simulink model "task_1"  (R2024a)
settings: Solver=VariableStepAuto  StartTime=0.0  StopTime=10  RelTol=1e-3
undefined symbols (not defined in the file): a0, a1, a2, idy, iy, k0, k1
settings Model: Creator=kit  LastModifiedBy=kit

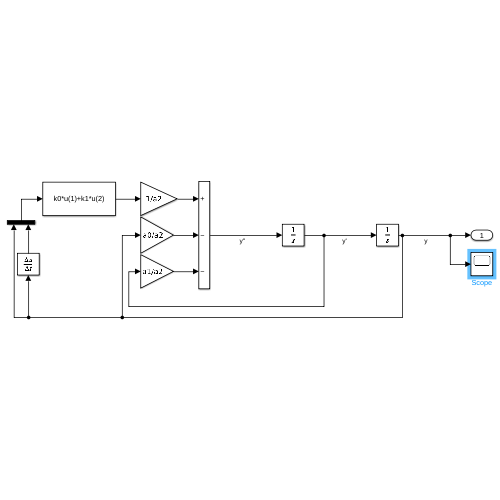
[thumbnail: Simulink's stored preview of the top-level diagram]
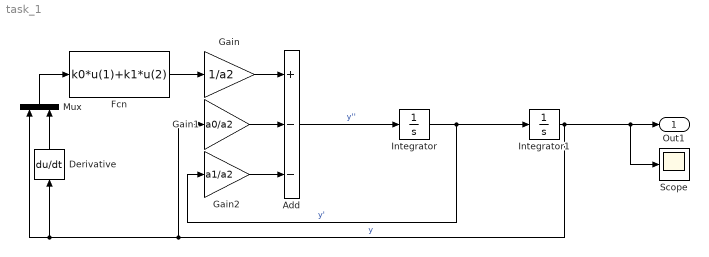
== system task_1 ==
  Add : Sum  Inputs=+--
  Derivative : Derivative
  Fcn : Fcn  Expr=k0*u(1)+k1*u(2)
  Gain : Gain  Gain=1/a2
  Gain1 : Gain  Gain=a0/a2
  Gain2 : Gain  Gain=a1/a2
  Integrator : Integrator  InitialCondition=idy
  Integrator1 : Integrator  InitialCondition=iy
  Mux : Mux  Inputs=2
  Scope : Scope
  Out1 : Outport
  wires:
  Fcn/1 -> Gain/1
  Gain/1 -> Add/1
  Gain2/1 -> Add/3
  Gain1/1 -> Add/2
  Add/1 -> Integrator/1  "y''"
  Integrator/1 -> Gain2/1, Integrator1/1  "y'"
  Integrator1/1 -> Gain1/1, Derivative/1, Mux/1, Scope/1, Out1/1  "y"
  Mux/1 -> Fcn/1
  Derivative/1 -> Mux/2
